simulink model "Harnes_Temp_Vary"  (R2018a)
settings: Solver=FixedStepDiscrete  StartTime=0.0  StopTime=inf  FixedStep=TimeSteps.ModelStep  RelTol=1e-6
undefined symbols (not defined in the file): Automatic_Test, Motor, Thermal
libraries: mciapi_libbrowser x1
settings Model: Creator=consul.marchionne  LastModifiedBy=PATILMP
settings DataIOCC: LimitDataPoints=on
settings OptimizationCC: LifeSpan=inf
settings DebuggingCC: SolverPrmCheckMsg=warning  SFUnexpectedBacktrackingDiag=warning  SFNoUnconditionalDefaultTransitionDiag=warning  SFExecutionAtInitializationDiag=none
settings HardwareCC: ProdBitPerPointer=32  ProdBitPerSizeT=32  ProdBitPerPtrDiffT=32  ProdLargestAtomicFloat=None  ProdIntDivRoundTo=Undefined  ProdEndianess=Unspecified  ProdWordSize=32  ProdHWDeviceType=32-bit Generic
settings ModelReferenceCC: UpdateModelReferenceTargets=IfOutOfDate  EnableRefExpFcnMdlSchedulingChecks=off  ModelReferenceNumInstancesAllowed=Single  ModelReferenceMinAlgLoopOccurrences=on  PropagateSignalLabelsOutOfModel=off
settings CodeAppCC: StateflowObjectComments=on
settings GRTTargetCC: TargetLangStandard=C89/C90 (ANSI)  GeneratePreprocessorConditionals=Disable all
settings ConfigComp: CovMetricSettings=dw  CovHtmlReporting=on  CovSaveCumulativeToWorkspaceVar=on  CovSaveSingleToWorkspaceVar=on  CovExternalEMLEnable=off  CovSFcnEnable=off

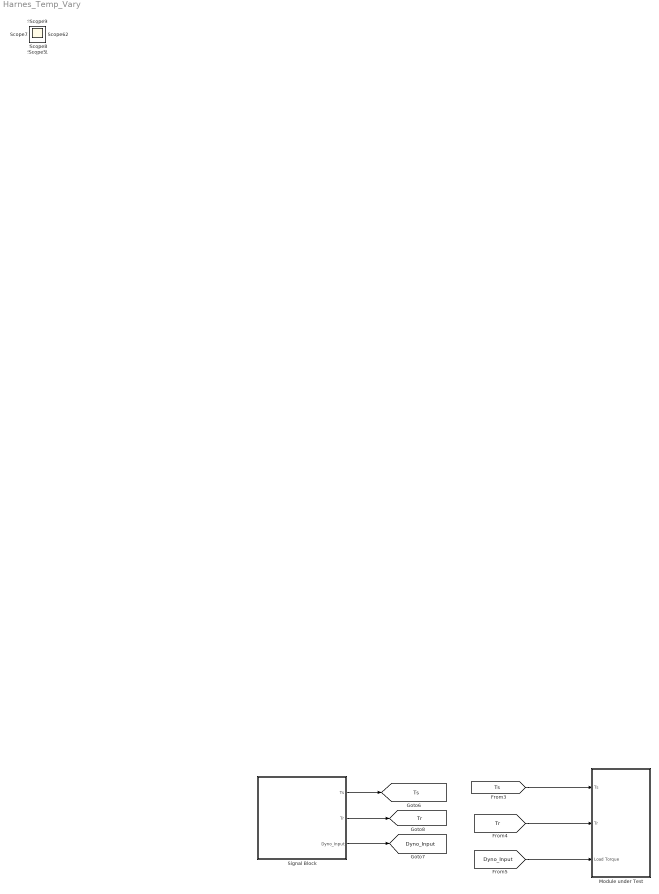
== system Harnes_Temp_Vary ==
  Module under Test : Subsystem  mask(Module under test){}
      mask help:
      | This harness block is used to test the exported block created in the simulation architecture.
      | User has to click on  look under mask and connect the three input ports such as Ts,Tr and Load Torque to the input port of exported block respectively.
  Signal Block : Subsystem
  Scope{,2..12} (12 alike) : Scope
  tag scope: Dyno_Input=global, Tr=global, Ts=global
  wires:
  Signal Block/2(Tr) -> [Tr]
  Signal Block/1(Ts) -> [Ts]
  Signal Block/3(Dyno_Input) -> [Dyno_Input]
  [Ts] -> Module under Test/1(Ts)
  [Tr] -> Module under Test/2(Tr)
  [Dyno_Input] -> Module under Test/3(Load Torque)

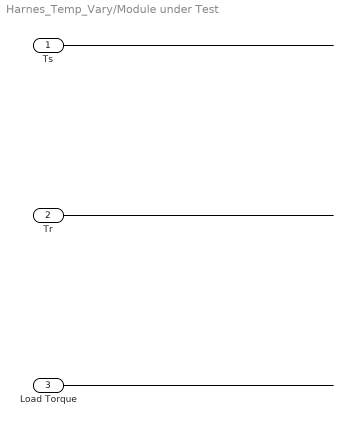
== system Harnes_Temp_Vary/Module under Test ==
  Ts : Inport
  Tr : Inport  Port=2
  Load Torque : Inport  Port=3
  wires:
  Ts/1 -> ?
  Tr/1 -> ?
  Load Torque/1 -> ?

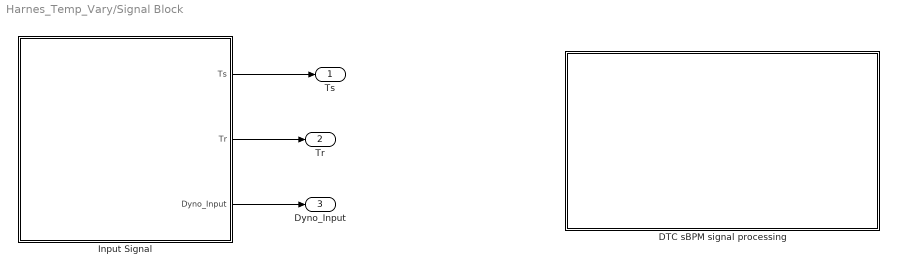
== system Harnes_Temp_Vary/Signal Block ==
  DTC sBPM signal processing : Subsystem
  Input Signal : Subsystem
  Ts : Outport
  Tr : Outport  Port=2
  Dyno_Input : Outport  Port=3
  wires:
  Input Signal/1(Ts) -> Ts/1
  Input Signal/2(Tr) -> Tr/1
  Input Signal/3(Dyno_Input) -> Dyno_Input/1

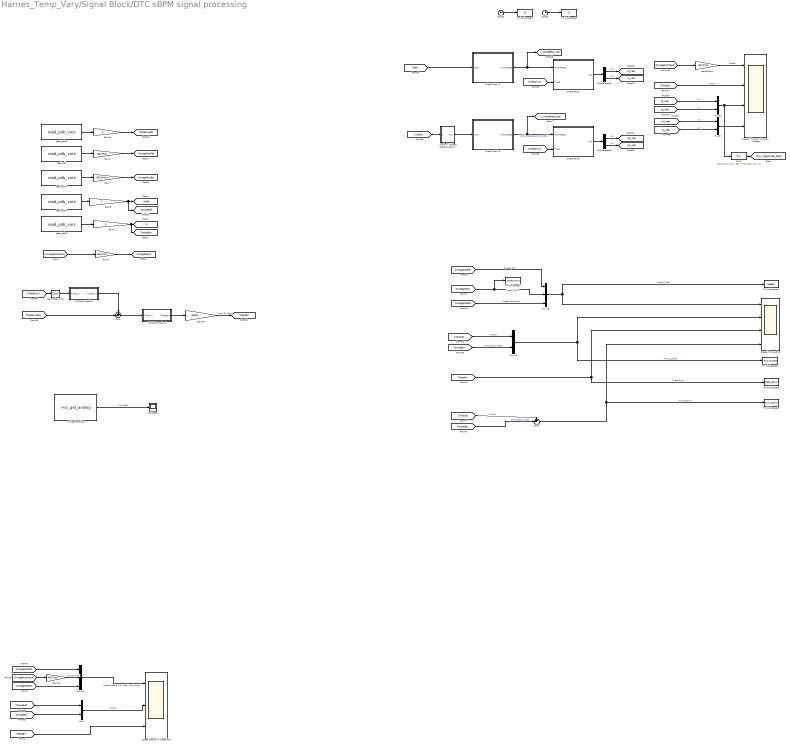
== system Harnes_Temp_Vary/Signal Block/DTC sBPM signal processing ==
  Bus Selector6 : BusSelector  OutputSignals=D,Q
  Bus Selector9 : BusSelector  OutputSignals=D,Q
  Clock2 : Clock
  Clock3 : Clock
  Direct  Clark  2 : MATLAB Function  TreatAsAtomicUnit=on  SystemSampleTime=SystemSampleTime  mask{SystemSampleTime=-1}
      mask prompts: SystemSampleTime "Simulink:blkprm_prompts:AllBlksSampleTime"
  Direct  Clark  3 : MATLAB Function  TreatAsAtomicUnit=on  SystemSampleTime=SystemSampleTime  mask{SystemSampleTime=-1}
      mask prompts: SystemSampleTime "Simulink:blkprm_prompts:AllBlksSampleTime"
  Direct Park2 : MATLAB Function  TreatAsAtomicUnit=on  SystemSampleTime=SystemSampleTime  mask{SystemSampleTime=-1}
      mask prompts: SystemSampleTime "Simulink:blkprm_prompts:AllBlksSampleTime"
  Direct Park3 : MATLAB Function  TreatAsAtomicUnit=on  SystemSampleTime=SystemSampleTime  mask{SystemSampleTime=-1}
      mask prompts: SystemSampleTime "Simulink:blkprm_prompts:AllBlksSampleTime"
  Fcn5 : Fcn  Expr=sqrt((0.0212*u(1)+0.0688)^2+(0.0299*u(2))^2)
  Gain15 : Gain  OutDataTypeStr=double  RndMeth=Zero
  Gain19 : Gain  Gain=180/pi
  Gain2 : Gain  Gain=60/(2*pi)  RndMeth=Round
  Gain22 : Gain  Gain=60/(2*pi)  RndMeth=Round
  Gain6 : Gain  Gain=60/(2*pi)  OutDataTypeStr=double  RndMeth=Zero
  Gain7 : Gain  Gain=60/(2*pi)/4  OutDataTypeStr=double  RndMeth=Zero
  Gain8 : Gain  OutDataTypeStr=double  RndMeth=Zero
  Gain9 : Gain  OutDataTypeStr=double  RndMeth=Zero
  MATLAB Function1 : MATLAB Function  TreatAsAtomicUnit=on
  MATLAB Function2 : MATLAB Function  TreatAsAtomicUnit=on
  MCI_State : Scope
  Mux{1,16,32,37} (4 alike) : Mux  Inputs=2
  Mux10 : Mux  Inputs=3
  Mux15 : Mux  Inputs=3
  Speed - Torque - Current - Voltage : Scope  NumInputPorts=4
  Speed Control + Theta Error : Scope  NumInputPorts=3
  Speed-Torque-Error : Scope  NumInputPorts=4
  Sum : Sum  Inputs=+-|
  Sum1 : Sum  Inputs=+-|
  To Workspace1 : ToWorkspace  VariableName=Speed  SaveFormat=Timeseries  SampleTime=-1
  To Workspace2 : ToWorkspace  VariableName=t2  SampleTime=-1
      settings: Save2DSignal=2-D array (concatenate along first dimension)
  To Workspace3 : ToWorkspace  VariableName=t3  SampleTime=-1
      settings: Save2DSignal=2-D array (concatenate along first dimension)
  To Workspace4 : ToWorkspace  VariableName=Torque_Data  SaveFormat=Timeseries  SampleTime=-1
  To Workspace5 : ToWorkspace  VariableName=Torque_Error  SaveFormat=Timeseries  SampleTime=-1
  To Workspace6 : ToWorkspace  VariableName=Theta_Error  SaveFormat=Timeseries  SampleTime=-1
  To Workspace7 : ToWorkspace  VariableName=Speed_Plant  SaveFormat=Timeseries  SampleTime=-1
  "Vpole -> Vphase reconstruction1" : MATLAB Function  TreatAsAtomicUnit=on
  Zero-Order Hold : ZeroOrderHold  SampleTime=0.000125
  mci_get_analog : S-Function  FunctionName=mci_get_analog  Parameters=read_data, choose_read_data  SFunctionDeploymentMode=off  EnableBusSupport=off  mask{choose_read_data=MCI_AI_INTERNAL_MCI_STATE, read_data=24}
      mask prompts: choose_read_data "Data to read"
      mask TypeOptions choose_read_data: MCI_AI_TARGET_SPEED_RPM_S16 | MCI_AI_SPEED_REFERENCE_RPM_S16 | MCI_AI_ACTUAL_SPEED_S16 | MCI_AI_SPEED_ERROR_RPM_S16 | MCI_AI_MEAN_SPEED_S16 | MCI_AI_RMS_MOTOR_CURRENT_S16 | MCI_AI_ACTIVE_POWER_S16 | MCI_AI_SHAFT_POWER_S16 | MCI_AI_MOTOR_TEMP_S16 | MCI_AI_STATOR_TEMP_S16 | MCI_AI_LOAD_TORQUE_S16 | MCI_AI_SHAFT_POSITION_DEG_S16 | MCI_AI_BUS_CURRENT_S16 | MCI_AI_BUS_VOLTAGE_S16 | MCI_AI_INVERTER_TEMP_S16 | MCI_AI_INVERTER_TEMP_RAW_DATA | MCI_AI_VOLTAGE_PHASE_A_S16 | MCI_AI_VOLTAGE_PHASE_B_S16 | MCI_AI_VOLTAGE_PHASE_C_S16 | MCI_AI_SPEED_LOOP_GAIN_TABLE_INDEX | MCI_AI_CURR_PHASE_A_S16 | MCI_AI_CURR_PHASE_B_S16 | MCI_AI_CURR_PHASE_C_S16 | MCI_AI_STATOR_RESISTANCE_S16 | MCI_AI_INTERNAL_MCI_STATE
      mask Callback read_data:
      | rd = get_param(gcb,'choose_read_data');
      | poenum = strcat('MCI_AI_TYPE.',rd);
      | i_32 = eval(['int32(' poenum ')']);
      | set_param(gcb,'read_data',int2str(i_32));
      mask Display:
      | disp = regexp(choose_read_data, 'MCI_AI_', 'split');
      | port_label('output', 1, disp{2});
  rad/s2Rpm1 : Gain  Gain=60/(2*pi)
  read_pdb : S-Function  FunctionName=read_pdb_vars  Parameters=vstring  SFunctionDeploymentMode=off  EnableBusSupport=off  mask{vstring=Mcl_IO.Speed_Rot_Ref}
      mask prompts: vstring "Variable to read"
      mask Display:
      | disp = vstring;
      | port_label('output', 1, disp);
  read_pdb1 : S-Function  FunctionName=read_pdb_vars  Parameters=vstring  SFunctionDeploymentMode=off  EnableBusSupport=off  mask{vstring=Mcl_Quantities.Speed_Rot}
      mask prompts: vstring "Variable to read"
      mask Display:
      | disp = vstring;
      | port_label('output', 1, disp);
  read_pdb2 : S-Function  FunctionName=read_pdb_vars  Parameters=vstring  SFunctionDeploymentMode=off  EnableBusSupport=off  mask{vstring=Mcl_Quantities.Torque_Ref}
      mask prompts: vstring "Variable to read"
      mask Display:
      | disp = vstring;
      | port_label('output', 1, disp);
  read_pdb3 : S-Function  FunctionName=read_pdb_vars  Parameters=vstring  SFunctionDeploymentMode=off  EnableBusSupport=off  mask{vstring=Mcl_Quantities.Torque}
      mask prompts: vstring "Variable to read"
      mask Display:
      | disp = vstring;
      | port_label('output', 1, disp);
  read_pdb8 : S-Function  FunctionName=read_pdb_vars  Parameters=vstring  SFunctionDeploymentMode=off  EnableBusSupport=off  mask{vstring=Mcl_Quantities.Rotor_Position}
      mask prompts: vstring "Variable to read"
      mask Display:
      | disp = vstring;
      | port_label('output', 1, disp);
  tag scope: I_AlphaBeta_real=global, Id_real=global, Iq=global, IqRef=global, Iq_real=global, OmegaMech=global, OmegaRotEst=global, OmegaRotRef=global, ThetaErr=global, ThetaFluxEst=global, TorqueEst=global, TorqueRef=global, V_AlphaBeta_real=global, Vd_real=global, Vq_real=global
  wires:
  [ThetaFlux] -> Zero-Order Hold/1
  MATLAB Function1/1(Theta_out) -> Sum/1
  Sum/1 -> MATLAB Function2/1(Theta_in)
  Gain19/1 -> [ThetaErr]  "Theta Err [deg]"
  MATLAB Function2/1(Theta_out) -> Gain19/1
  Zero-Order Hold/1 -> MATLAB Function1/1(Theta_in)
  [ThetaFluxEst] -> Sum/2
  Bus Selector6/1 -> [Id_real]  "<D>"
  [Vpole] -> "Vpole -> Vphase reconstruction1"/1(Vpole)
  [Vq_real] -> Mux37/2  "Vq"
  Bus Selector6/2 -> [Iq_real]  "<Q>"
  "Vpole -> Vphase reconstruction1"/1(Vout) -> Direct  Clark  3/1(Xabc)
  [ThetaFlux] -> Direct Park3/2(Theta)
  Mux32/1 -> Fcn5/1, Speed - Torque - Current - Voltage/3
  Direct Park2/1(Xdq) -> Bus Selector6/1
  Clock2/1 -> To Workspace2/1
  [Iq_real] -> Mux32/2  "Iq"
  rad/s2Rpm1/1 -> Speed - Torque - Current - Voltage/1  "Speed"
  Mux37/1 -> Speed - Torque - Current - Voltage/4
  Clock3/1 -> To Workspace3/1
  [Iabc] -> Direct  Clark  2/1(Xabc)
  Bus Selector9/1 -> [Vd_real]  "<D>"
  [ThetaFlux] -> Direct Park2/2(Theta)
  [Torque] -> Speed - Torque - Current - Voltage/2  "Torque"
  [Id_real] -> Mux32/1  "Id"
  [Vd_real] -> Mux37/1  "Vd"
  Bus Selector9/2 -> [Vq_real]  "<Q>"
  Direct  Clark  3/1(XAlphaBeta) -> Direct Park3/1(XAlphaBeta), [V_AlphaBeta_real]  "Valpha_Beta_reconstructed"
  Direct Park3/1(Xdq) -> Bus Selector9/1
  Direct  Clark  2/1(XAlphaBeta) -> [I_AlphaBeta_real], Direct Park2/1(XAlphaBeta)
  [OmegaRotMech] -> rad/s2Rpm1/1
  Gain8/1 -> [TorqueRef], [IqRef]
  Gain9/1 -> [TorqueEst], [Iq]
  read_pdb/1 -> Gain6/1
  read_pdb8/1 -> Gain15/1
  Gain15/1 -> [ThetaFluxEst]
  read_pdb3/1 -> Gain9/1
  read_pdb2/1 -> Gain8/1
  Gain6/1 -> [OmegaRotRef]
  read_pdb1/1 -> Gain7/1
  Gain7/1 -> [OmegaRotEst]
  [TorqueEst] -> Mux1/2
  [TorqueRef] -> Mux1/1
  Mux1/1 -> Speed Control + Theta Error/2  "Torque"
  mci_get_analog/1 -> MCI_State/1  "MCI_State"
  Fcn5/1 -> [Flux_Magnitude_Real]
  Mux15/1 -> Speed-Torque-Error/1, To Workspace1/1  "Speed_Data"
  [TorqueEst] -> Sum1/2  "Torque_estimated"
  [TorqueEst] -> Mux16/2  "Torque_estimated"
  [Torque] -> Mux16/1  "Torque"
  Sum1/1 -> Speed-Torque-Error/4, To Workspace5/1  "Torque Error"
  [OmegaRotEst] -> Mux15/3  "Speed Estimated"
  [OmegaMech] -> To Workspace7/1, Mux15/2  "Speed Plant"
  [Torque] -> Sum1/1  "Torque"
  Mux16/1 -> To Workspace4/1, Speed-Torque-Error/2  "Torque_Data"
  [ThetaErr] -> To Workspace6/1, Speed-Torque-Error/3  "Theta Error"
  [OmegaRotRef] -> Mux15/1  "Speed_Ref"
  [OmegaRotEst] -> Mux10/3
  Gain22/1 -> Mux10/2  "Speed Real"
  [OmegaRotRef] -> Mux10/1
  Mux10/1 -> Speed Control + Theta Error/1  "Speed Reference - Real - Estimated"
  [OmegaRotMech] -> Gain22/1
  [ThetaErr] -> Speed Control + Theta Error/3
  Gain2/1 -> [OmegaMech]
  [OmegaRotMech] -> Gain2/1

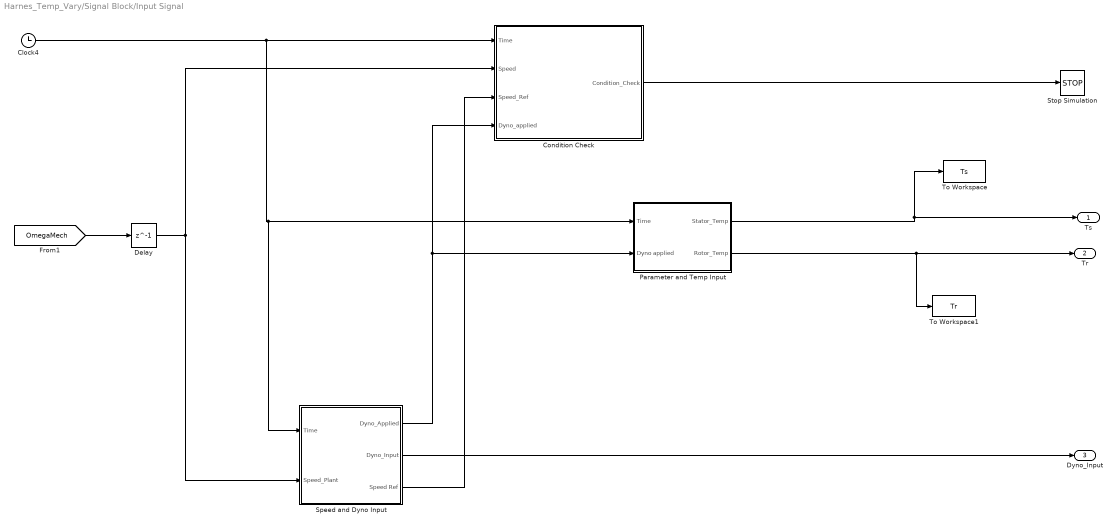
== system Harnes_Temp_Vary/Signal Block/Input Signal ==
  Clock4 : Clock
  Condition Check : MATLAB Function  TreatAsAtomicUnit=on  mask(Condition Check){Speed_Tolerance=Automatic_Test.Speed_Tolerance, Para_time_check=Automatic_Test.Para_time_check}
      mask prompts: Speed_Tolerance "Speed Tolerance Value"; Para_time_check "Parameter Time Check"
      mask help: This function block keeps check on failurity of the Test.
  Delay : Delay  DelayLength=1
  Parameter and Temp Input : Subsystem
  Speed and Dyno Input : Subsystem
  Stop Simulation : Stop
  To Workspace : ToWorkspace  VariableName=Ts  SaveFormat=Structure  SampleTime=-1
  To Workspace1 : ToWorkspace  VariableName=Tr  SaveFormat=Structure  SampleTime=-1
  Ts : Outport
  Tr : Outport  Port=2
  Dyno_Input : Outport  Port=3
  wires:
  Speed and Dyno Input/1(Dyno_Applied) -> Condition Check/4(Dyno_applied), Parameter and Temp Input/2(Dyno applied)
  Speed and Dyno Input/3(Speed Ref) -> Condition Check/3(Speed_Ref)
  Delay/1 -> Condition Check/2(Speed), Speed and Dyno Input/2(Speed_Plant)
  Clock4/1 -> Speed and Dyno Input/1(Time), Parameter and Temp Input/1(Time), Condition Check/1(Time)
  [OmegaMech] -> Delay/1
  Condition Check/1(Condition_Check) -> Stop Simulation/1
  Speed and Dyno Input/2(Dyno_Input) -> Dyno_Input/1
  Parameter and Temp Input/1(Stator_Temp) -> To Workspace/1, Ts/1
  Parameter and Temp Input/2(Rotor_Temp) -> To Workspace1/1, Tr/1

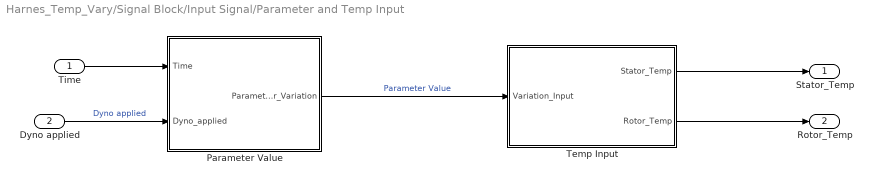
== system Harnes_Temp_Vary/Signal Block/Input Signal/Parameter and Temp Input ==
  Time : Inport
  Dyno applied : Inport  Port=2
  Parameter Value : MATLAB Function  TreatAsAtomicUnit=on  mask(Parameter Value){init_value=Motor.Electrical.Rs_a_Ref, Para_time_check=Automatic_Test.Para_time_check, Percentage_Variation=Automatic_Test.Percentage_Variation}
      mask prompts: init_value "Intital Value"; Para_time_check "Time_Check"; Percentage_Variation "Percentage Variation"
      mask help: This Matlab function block is used to input the parameter variation signal.
  Temp Input : MATLAB Function  TreatAsAtomicUnit=on  mask(Temp Input){Init_Value=Motor.Electrical.Rs_a_Ref, Temp_Ref=Motor.Mechanical.Rs_Temperature_Ref, alpha=Motor.Electrical.alpha_s, flag=strcmp(Automatic_Test.parameter_var,'Rs')}
      mask prompts: Init_Value "Parameter Intial Value"; Temp_Ref "Temperature Referance"; flag "Selection of Test"
      mask help: This Matlab function block is used to input temperature to stator and Rotor.
  Stator_Temp : Outport
  Rotor_Temp : Outport  Port=2
  wires:
  Parameter Value/1(Parameter_Variation) -> Temp Input/1(Variation_Input)  "Parameter Value"
  Time/1 -> Parameter Value/1(Time)
  Dyno applied/1 -> Parameter Value/2(Dyno_applied)  "Dyno applied"
  Temp Input/1(Stator_Temp) -> Stator_Temp/1
  Temp Input/2(Rotor_Temp) -> Rotor_Temp/1

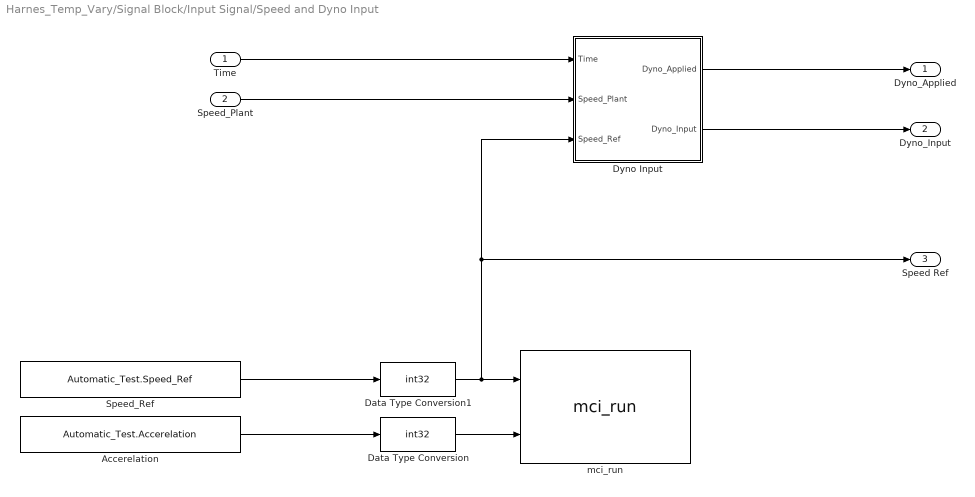
== system Harnes_Temp_Vary/Signal Block/Input Signal/Speed and Dyno Input ==
  Time : Inport
  Speed_Plant : Inport  Port=2
  Accerelation : Constant  Value=Automatic_Test.Accerelation
  Data Type Conversion : DataTypeConversion  OutDataTypeStr=int32
  Data Type Conversion1 : DataTypeConversion  OutDataTypeStr=int32
  Dyno Input : Subsystem
      mask Display:
      | port_label('Input',1,'Time');
      | port_label('Input',2,'Speed_Plant');
      | port_label('Input',3,'Speed_Ref');
      | port_label('output',1,'Dyno_Applied');
      | port_label('output',2,'Dyno_Input');
  Speed_Ref : Constant  Value=Automatic_Test.Speed_Ref
  mci_run : mciapi_libbrowser/mci_run  SFunctionModules=''
      settings: SourceProductName=Sim Arch
  Dyno_Applied : Outport
  Dyno_Input : Outport  Port=2
  Speed Ref : Outport  Port=3
  wires:
  Accerelation/1 -> Data Type Conversion/1
  Speed_Ref/1 -> Data Type Conversion1/1
  Data Type Conversion/1 -> mci_run/2
  Time/1 -> Dyno Input/1(Time)
  Speed_Plant/1 -> Dyno Input/2(Speed_Plant)
  Dyno Input/2(Dyno_Input) -> Dyno_Input/1
  Dyno Input/1(Dyno_Applied) -> Dyno_Applied/1
  Data Type Conversion1/1 -> Dyno Input/3(Speed_Ref), Speed Ref/1, mci_run/1

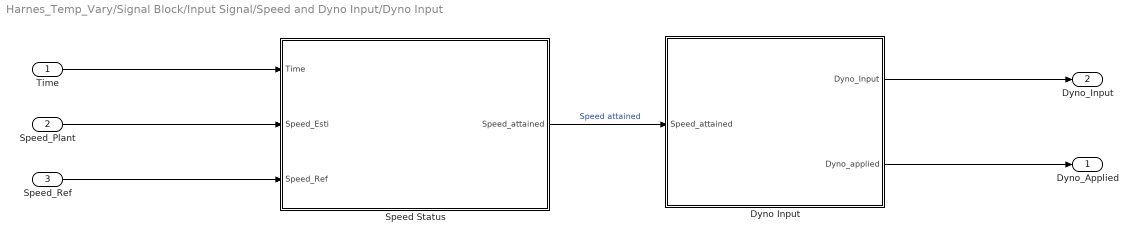
== system Harnes_Temp_Vary/Signal Block/Input Signal/Speed and Dyno Input/Dyno Input ==
  Time : Inport
  Speed_Plant : Inport  Port=2
  Speed_Ref : Inport  Port=3
  Dyno Input : MATLAB Function  TreatAsAtomicUnit=on  mask(Dyno Input){Dyno_Load=Automatic_Test.Dyno_Load, Dyno_Step_Size=Automatic_Test.Dyno_Step_Size}
      mask prompts: Dyno_Load "Dyno Load Value"; Dyno_Step_Size "Dyno Step Size"
      mask help: This Matlab function block is used to input Dyno load.
  Speed Status : MATLAB Function  TreatAsAtomicUnit=on  mask(Speed Status){Status_Tolerance=Automatic_Test.Status_Tolerance, Status_Time_Check=Automatic_Test.Status_Time_Check}
      mask prompts: Status_Tolerance "Status Tolerance"; Status_Time_Check "Status Time Check"
      mask help: This Matlab function block is used to get the status of reference and estimated speed.
  Dyno_Applied : Outport
  Dyno_Input : Outport  Port=2
  wires:
  Speed_Ref/1 -> Speed Status/3(Speed_Ref)
  Time/1 -> Speed Status/1(Time)
  Speed_Plant/1 -> Speed Status/2(Speed_Esti)
  Speed Status/1(Speed_attained) -> Dyno Input/1(Speed_attained)  "Speed attained"
  Dyno Input/1(Dyno_Input) -> Dyno_Input/1
  Dyno Input/2(Dyno_applied) -> Dyno_Applied/1

== matlab function Harnes_Temp_Vary/Signal Block/DTC sBPM signal processing/Direct  Clark  2 ==
  data: XAlphaBeta output Bus: XAlphaBetaBus; Xabc input Bus: XabcBus
function XAlphaBeta = DirectClark(Xabc)

XAlphaBeta.Alpha = Xabc.A;
XAlphaBeta.Beta =  sqrt(3)/3*(Xabc.A+2*Xabc.B);

== matlab function Harnes_Temp_Vary/Signal Block/DTC sBPM signal processing/Direct  Clark  3 ==
  data: XAlphaBeta output Bus: XAlphaBetaBus; Xabc input Bus: XabcBus
function XAlphaBeta = DirectClark(Xabc)

XAlphaBeta.Alpha = Xabc.A;
XAlphaBeta.Beta =  sqrt(3)/3*(Xabc.A+2*Xabc.B);

== matlab function Harnes_Temp_Vary/Signal Block/DTC sBPM signal processing/Direct Park2 ==
  data: XAlphaBeta input Bus: XAlphaBetaBus; Xdq output Bus: XdqBus; Theta input
function Xdq = DirectPark(XAlphaBeta,Theta)

Xdq.D  =  XAlphaBeta.Alpha*cos(Theta) + XAlphaBeta.Beta*sin(Theta);
Xdq.Q  = -XAlphaBeta.Alpha*sin(Theta) + XAlphaBeta.Beta*cos(Theta);

== matlab function Harnes_Temp_Vary/Signal Block/DTC sBPM signal processing/Direct Park3 ==
  data: XAlphaBeta input Bus: XAlphaBetaBus; Xdq output Bus: XdqBus; Theta input
function Xdq = DirectPark(XAlphaBeta,Theta)

Xdq.D  =  XAlphaBeta.Alpha*cos(Theta) + XAlphaBeta.Beta*sin(Theta);
Xdq.Q  = -XAlphaBeta.Alpha*sin(Theta) + XAlphaBeta.Beta*cos(Theta);

== matlab function Harnes_Temp_Vary/Signal Block/DTC sBPM signal processing/MATLAB Function1 ==
  data: Theta_in input; Theta_out output
function Theta_out = fcn(Theta_in)
%#codegen

if(Theta_in > pi)||(Theta_in < -pi)
    
    Resto_pi =  mod(Theta_in, pi);
    Resto_2pi =  mod(Theta_in, 2*pi);
    
    
    if(Resto_pi ~= Resto_2pi)
    Theta_out = -pi+Resto_pi;
    else
    Theta_out = Resto_pi;    
    end
 
else
    
    Theta_out = Theta_in;
    
end

== matlab function Harnes_Temp_Vary/Signal Block/DTC sBPM signal processing/MATLAB Function2 ==
  data: Theta_in input; Theta_out output
function Theta_out = fcn(Theta_in)
%#codegen

if(Theta_in > pi)||(Theta_in < -pi)
    
    Resto_pi =  mod(Theta_in, pi);
    Resto_2pi =  mod(Theta_in, 2*pi);
    
    
    if(Resto_pi ~= Resto_2pi)
    Theta_out = -pi+Resto_pi;
    else
    Theta_out = Resto_pi;    
    end
 
else
    
    Theta_out = Theta_in;
    
end

== matlab function Harnes_Temp_Vary/Signal Block/DTC sBPM signal processing/Vpole -> Vphase reconstruction1 ==
  data: Vpole input Bus: XabcBus size=1; Vout output Bus: XabcBus
function Vout   = Vrec2(Vpole)

Va = Vpole.A;
Vb = Vpole.B;
Vc = Vpole.C;

Vn = (Va + Vb + Vc)/3;

Vphase.A = Va - Vn;
Vphase.B = Vb - Vn;
Vphase.C = Vc - Vn;

Vline.A = Va - Vb;  % Vab
Vline.B = Vb - Vc;  % Vbc
Vline.C = Vc - Va;  % Vca

Vout = Vphase;
end

== matlab function Harnes_Temp_Vary/Signal Block/Input Signal/Condition Check ==
  data: Time input; Speed input; Speed_Ref input; Condition_Check output; Dyno_applied input; Speed_Tolerance parameter; Para_time_check parameter
function Condition_Check = fcn(Time,Speed,Speed_Ref,Dyno_applied, Speed_Tolerance,Para_time_check)
persistent old_value
if isempty(old_value)
    old_value=0;
end

ST=Speed_Tolerance/100;
Limit=Speed_Ref*ST;
Delta_Speed=abs(Speed-Speed_Ref);


Condition_Check = 0;

if Dyno_applied==1
    if (Delta_Speed > Limit)
        if ((Time-old_value)>0.3*Para_time_check)
            Condition_Check = 1; 
        end
    else
        old_value = Time;
    end
end


%Automatic_Test.Dyno_Load_Vector=0.5;%[0.5;0.85;1.28];

== matlab function Harnes_Temp_Vary/Signal Block/Input Signal/Parameter and Temp Input/Parameter Value ==
  data: Time input; Dyno_applied input; Parameter_Variation output; Para_time_check parameter; Percentage_Variation parameter; init_value parameter

function Parameter_Variation   = fcn(Time,Dyno_applied,Para_time_check, Percentage_Variation,init_value)
persistent old_value
persistent old_time
% step=Percentage/100;  % later put as parameter



step=(Percentage_Variation/100)*init_value;


if isempty(old_value)
    old_value=init_value;
end
   
if isempty(old_time)
    old_time=0;
end

if Dyno_applied==1
    if ((Time-old_time)> Para_time_check)
        old_time=Time;
        old_value= old_value+step;
       
    end
    
else
    old_time=Time;
end
    

Parameter_Variation =old_value;

== matlab function Harnes_Temp_Vary/Signal Block/Input Signal/Parameter and Temp Input/Temp Input ==
  data: Variation_Input input; Init_Value parameter; Temp_Ref parameter; Stator_Temp output; alpha parameter; Thermal parameter; Rotor_Temp output; flag parameter
function [Stator_Temp,Rotor_Temp] = fcn(Variation_Input,Init_Value,Temp_Ref,alpha,Thermal,flag) %fcn(Input,Init_Value, Temp_Ref,alpha)
Stator_Temp=0;
Rotor_Temp=0;
%......Calculation of Temperature T with corrosponding change in Parameter....%

 Temp=(Variation_Input+Init_Value*(alpha*Temp_Ref-1))/(Init_Value*alpha);
 
if(flag==1)
Stator_Temp=Temp; 
Rotor_Temp= Thermal.Trotor;
 end
if(flag==0)
 Rotor_Temp=Temp; 
 Stator_Temp=Thermal.Tstator;
end









% 
% function [Stator_Temp,Rotor_Temp] = fcn(Input,Init_Value,Temp_Ref,alpha,Thermal,flag) %fcn(Input,Init_Value, Temp_Ref,alpha)
% Stator_Temp=0;
% Rotor_Temp=0;
% %......Calculation of Temperature T with corrosponding change in Parameter....%
% 
%  Temp=(Input+Init_Value*(alpha*Temp_Ref-1))/(Init_Value*alpha);
%  
% if(flag==1)
% Stator_Temp=Temp; 
% Rotor_Temp= Thermal.Trotor;
%  end
% if(flag==0)
%  Rotor_Temp=Temp; 
%  Stator_Temp=Thermal.Tstator;
% end

== matlab function Harnes_Temp_Vary/Signal Block/Input Signal/Speed and Dyno Input/Dyno Input/Dyno Input ==
  data: Dyno_Input output; Speed_attained input; Dyno_applied output; Dyno_Load parameter; Dyno_Step_Size parameter
function [Dyno_Input,Dyno_applied] = fcn(Speed_attained, Dyno_Load,Dyno_Step_Size )
persistent old_value
 


init_value=0;
Dyno_applied=0;

if isempty(old_value)
    old_value=init_value;
    
end

if Speed_attained==1
    old_value=Dyno_Step_Size+old_value;
    
     if old_value>Dyno_Load
         
         old_value=Dyno_Load;
         Dyno_applied=1;
    end 
end

Dyno_Input=old_value;;

== matlab function Harnes_Temp_Vary/Signal Block/Input Signal/Speed and Dyno Input/Dyno Input/Speed Status ==
  data: Speed_attained output; Time input; Speed_Esti input; Speed_Ref input; Status_Tolerance parameter; Status_Time_Check parameter
function Speed_attained = fcn(Time,Speed_Esti,Speed_Ref,Status_Tolerance,Status_Time_Check)
persistent t_old
persistent flag


if isempty(t_old)
    t_old =0;
end

if isempty(flag)
    flag = 0;
end

if abs(Speed_Ref- Speed_Esti)<(Status_Tolerance*Speed_Ref)
   flag = 1;
end

if flag == 0
    t_old = Time;
end

if (Time-t_old)>Status_Time_Check
    Speed_attained = 1;
else
    Speed_attained = 0;
end
